simulink model "pitch_loop"  (Simulink 7.4)
settings: Solver=ode45  StartTime=0.0  StopTime=30  RelTol=1e-3
values from neighbouring files (symbols this model uses):
  a_theta1 = den(2)    [computeGains.m]    (also in compute_tf_model.m = -rho*Va_trim^2 * cbar^2 * S_wing /(4*P.Jy) * P.C_M_q)
  a_theta2 = num(3)    [computeGains.m]    (also in compute_tf_model.m = -rho*Va_trim^2*cbar*S_wing/2/P.Jy*C_M_alpha)
  a_theta3 = rho*Va_trim^2*cbar*S_wing/2/P.Jy*C_M_delta_e    [compute_tf_model.m]
  delta_e_max = P.delta_e_max    [computeGains.m]
  P = varargin{5}    [my_mav_dynamics.m]
undefined symbols (not defined in the file or in its folder): K_theta_DC, theta_max
settings Model: Creator=beard  LastModifiedBy=beard

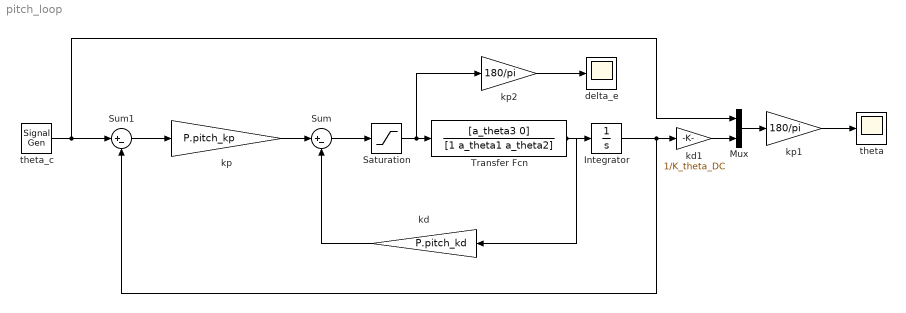
== system pitch_loop ==
  Integrator : Integrator
  Mux : Mux  Inputs=2
  Saturation : Saturate  UpperLimit=delta_e_max  LowerLimit=-delta_e_max  OutDataType=fixdt(1, 16)  OutScaling=2^0
  Sum : Sum  Inputs=|+-  OutDataType=fixdt(1, 16)  OutScaling=2^0
  Sum1 : Sum  Inputs=|+-  OutDataType=fixdt(1, 16)  OutScaling=2^0
  Transfer Fcn : TransferFcn  Numerator=[a_theta3 0]  Denominator=[1 a_theta1 a_theta2]
  delta_e : Scope
      settings: TimeRange=30  YMin=-100  YMax=100
  kd : Gain  Gain=P.pitch_kd  ParameterDataType=fixdt(1, 16)  ParameterScaling=2^0  OutDataType=fixdt(1, 16)  OutScaling=2^0
  kd1 : Gain  Gain=1/K_theta_DC  ParameterDataType=fixdt(1, 16)  ParameterScaling=2^0  OutDataType=fixdt(1, 16)  OutScaling=2^0
  kp : Gain  Gain=P.pitch_kp  ParameterDataType=fixdt(1, 16)  ParameterScaling=2^0  OutDataType=fixdt(1, 16)  OutScaling=2^0
  kp1 : Gain  Gain=180/pi  ParameterDataType=fixdt(1, 16)  ParameterScaling=2^0  OutDataType=fixdt(1, 16)  OutScaling=2^0
  kp2 : Gain  Gain=180/pi  ParameterDataType=fixdt(1, 16)  ParameterScaling=2^0  OutDataType=fixdt(1, 16)  OutScaling=2^0
  theta : Scope
      settings: TimeRange=30  YMin=-15  YMax=15
  theta_c : SignalGenerator  WaveForm=square  Amplitude=theta_max  Frequency=.05
  wires:
  Transfer Fcn/1 -> Integrator/1, kd/1
  Saturation/1 -> Transfer Fcn/1, kp2/1
  Sum/1 -> Saturation/1
  Sum1/1 -> kp/1
  Integrator/1 -> Sum1/2, kd1/1
  theta_c/1 -> Sum1/1, Mux/1
  kp1/1 -> theta/1
  Mux/1 -> kp1/1
  kp2/1 -> delta_e/1
  kp/1 -> Sum/1
  kd/1 -> Sum/2
  kd1/1 -> Mux/2
